simulink model "lab3_prob2_rd5"  (R2024a)
settings: Solver=VariableStepAuto  StartTime=0.0  StopTime=20  RelTol=1e-3
values from neighbouring files (symbols this model uses):
  G1H2G2G3G4H3_den = conv(TF_H2G2G3G4H3_den, G1G4_den)    [Problem2_Aldovino_Bejasa.m]
  G1H2G2G3G4H3_num = conv(TF_H2G2G3G4H3_num, G1G4_num)    [Problem2_Aldovino_Bejasa.m]
  H_den1 = [1 0]    [Problem2_Aldovino_Bejasa.m]
  H_num1 = [1]    [Problem2_Aldovino_Bejasa.m]
settings Model: Creator=HUAWEI  LastModifiedBy=HUAWEI

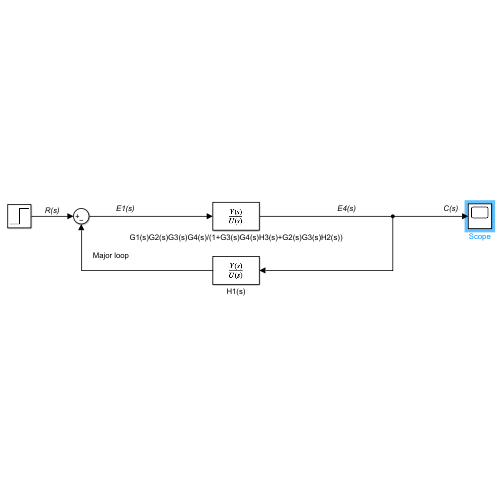
[thumbnail: Simulink's stored preview of the top-level diagram]
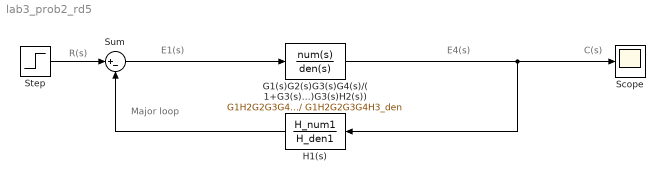
== system lab3_prob2_rd5 ==
  note: Major loop
  note: C(s)
  note: E4(s)
  note: E1(s)
  note: R(s)
  G1(s)G2(s)G3(s)G4(s)/(1+G3(s)G4(s)H3(s)+G2(s)G3(s)H2(s)) : TransferFcn  Numerator=G1H2G2G3G4H3_num  Denominator=G1H2G2G3G4H3_den
  H1(s) : TransferFcn  Numerator=H_num1  Denominator=H_den1
  Scope : Scope
  Step : Step  Time=0  SampleTime=0
  Sum : Sum  Inputs=|+-
  wires:
  H1(s)/1 -> Sum/2
  Step/1 -> Sum/1
  Sum/1 -> G1(s)G2(s)G3(s)G4(s)/(1+G3(s)G4(s)H3(s)+G2(s)G3(s)H2(s))/1
  G1(s)G2(s)G3(s)G4(s)/(1+G3(s)G4(s)H3(s)+G2(s)G3(s)H2(s))/1 -> H1(s)/1, Scope/1
